simulink model "GUI_Simulaton"  (R2022b)
settings: Solver=ode1  StartTime=0.0  StopTime=3  FixedStep=20/(0.5*PWMclock)  RelTol=1e-3
InitFcn:
  | addpath('..\Library_Subsystems')
  | 
  | load('PWMLookUp.mat')
  | load('SimDefaultParam.mat')
  | 
  | samplerate = 10e-3;
  | samplerate_serial = 100e-3;
  | samplerate_udp = 100e-3;
  | 
  | fsw = 10000;
  | 
  | PWMclock = 100e6;
  | period = PWMclock/fsw/2;
model workspace (MAT data in the model file):
  DPWM0 = Simulink.Parameter
  DPWM0.Value.Du = [0.75 0.752642797452 0.755257258329 0.757843284196 0.760400777693 0.762929642529 0.765429783496 0.767901106464 0.77034351839 0.772756927317 0.775141242383 0.77749637382 ... (1024 elements, 1024x1)]
  DPWM0.Value.Dusec = [-0.5 -0.5 -0.5 -0.5 -0.5 -0.5 -0.5 -0.5 -0.5 -0.5 -0.5 -0.5 ... (1024 elements, 1024x1)]
  DPWM0.Value.Duclamp = [0 0 0 0 0 0 0 0 0 0 0 0 ... (1024 elements, 1024x1)]
  DPWM0.Value.Dv = [0 0.00531383198086 0.0106274638989 0.015940695699 0.0212533273409 0.0265651588071 0.03187599011 0.0371856212999 0.0424938524722 0.0478004837749 0.0531053154165 0.0584081476729 ... (1024 elements, 1024x1)]
  DPWM0.Value.Dvsec = [-0.5 -0.5 -0.5 -0.5 -0.5 -0.5 -0.5 -0.5 -0.5 -0.5 -0.5 -0.5 ... (1024 elements, 1024x1)]
  DPWM0.Value.Dvclamp = [0 0 0 0 0 0 0 0 0 0 0 0 ... (1024 elements, 1024x1)]
  DPWM0.Value.Dw = [0 0 0 0 0 0 0 0 0 0 0 0 ... (1024 elements, 1024x1)]
  DPWM0.Value.Dwsec = [-0.5 -0.5 -0.5 -0.5 -0.5 -0.5 -0.5 -0.5 -0.5 -0.5 -0.5 -0.5 ... (1024 elements, 1024x1)]
  DPWM0.Value.Dwclamp = [2 2 2 2 2 2 2 2 2 2 2 2 ... (1024 elements, 1024x1)]
  DPWM0.Value.Dufi = [12288 12331 12374 12417 12458 12500 12541 12581 12621 12661 12700 12739 ... (1024 elements, 1024x1)]
  DPWM0.Value.Dusecfi = [-8192 -8192 -8192 -8192 -8192 -8192 -8192 -8192 -8192 -8192 -8192 -8192 ... (1024 elements, 1024x1)]
  DPWM0.Value.Dvfi = [0 87 174 261 348 435 522 609 696 783 870 957 ... (1024 elements, 1024x1)]
  DPWM0.Value.Dvsecfi = [-8192 -8192 -8192 -8192 -8192 -8192 -8192 -8192 -8192 -8192 -8192 -8192 ... (1024 elements, 1024x1)]
  DPWM0.Value.Dwfi = [0 0 0 0 0 0 0 0 0 0 0 0 ... (1024 elements, 1024x1)]
  DPWM0.Value.Dwsecfi = [-8192 -8192 -8192 -8192 -8192 -8192 -8192 -8192 -8192 -8192 -8192 -8192 ... (1024 elements, 1024x1)]
  DPWM0.DataType = 'struct'
  DPWM0.Complexity = 'real'
  DPWM0.Dimensions = [1 1]
  DPWM1.Duclamp = [1 1 1 1 1 1 1 1 1 1 1 1 ... (1024 elements, 1024x1)]
  DPWM1.Dvclamp = [0 0 0 0 0 0 0 0 0 0 0 0 ... (1024 elements, 1024x1)]
  DPWM1.Dwclamp = [0 0 0 0 0 0 0 0 0 0 0 0 ... (1024 elements, 1024x1)]
  DPWM1.Dufi = [0 0 0 0 0 0 0 0 0 0 0 0 ... (1024 elements, 1024x1)]
  DPWM1.Dusecfi = [8192 8192 8192 8192 8192 8192 8192 8192 8192 8192 8192 8192 ... (1024 elements, 1024x1)]
  DPWM1.Dvfi = [-12288 -12244 -12200 -12155 -12110 -12065 -12019 -11972 -11925 -11878 -11830 -11782 ... (1024 elements, 1024x1)]
  DPWM1.Dvsecfi = [8192 8192 8192 8192 8192 8192 8192 8192 8192 8192 8192 8192 ... (1024 elements, 1024x1)]
  DPWM1.Dwfi = [-12288 -12331 -12374 -12417 -12458 -12500 -12541 -12581 -12621 -12661 -12700 -12739 ... (1024 elements, 1024x1)]
  DPWM1.Dwsecfi = [8192 8192 8192 8192 8192 8192 8192 8192 8192 8192 8192 8192 ... (1024 elements, 1024x1)]
  DPWM2.Duclamp = [1 1 1 1 1 1 1 1 1 1 1 1 ... (1024 elements, 1024x1)]
  DPWM2.Dvclamp = [0 0 0 0 0 0 0 0 0 0 0 0 ... (1024 elements, 1024x1)]
  DPWM2.Dwclamp = [0 0 0 0 0 0 0 0 0 0 0 0 ... (1024 elements, 1024x1)]
  DPWM2.Dufi = [0 0 0 0 0 0 0 0 0 0 0 0 ... (1024 elements, 1024x1)]
  DPWM2.Dusecfi = [8192 8192 8192 8192 8192 8192 8192 8192 8192 8192 8192 8192 ... (1024 elements, 1024x1)]
  DPWM2.Dvfi = [-12288 -12244 -12200 -12155 -12110 -12065 -12019 -11972 -11925 -11878 -11830 -11782 ... (1024 elements, 1024x1)]
  DPWM2.Dvsecfi = [8192 8192 8192 8192 8192 8192 8192 8192 8192 8192 8192 8192 ... (1024 elements, 1024x1)]
  DPWM2.Dwfi = [-12288 -12331 -12374 -12417 -12458 -12500 -12541 -12581 -12621 -12661 -12700 -12739 ... (1024 elements, 1024x1)]
  DPWM2.Dwsecfi = [8192 8192 8192 8192 8192 8192 8192 8192 8192 8192 8192 8192 ... (1024 elements, 1024x1)]
  DPWM3.Duclamp = [0 0 0 0 0 0 0 0 0 0 0 0 ... (1024 elements, 1024x1)]
  DPWM3.Dvclamp = [0 0 0 0 0 0 0 0 0 0 0 0 ... (1024 elements, 1024x1)]
  DPWM3.Dwclamp = [2 2 2 2 2 2 2 2 2 2 2 2 ... (1024 elements, 1024x1)]
  DPWM3.Dufi = [12288 12331 12374 12417 12458 12500 12541 12581 12621 12661 12700 12739 ... (1024 elements, 1024x1)]
  DPWM3.Dusecfi = [-8192 -8192 -8192 -8192 -8192 -8192 -8192 -8192 -8192 -8192 -8192 -8192 ... (1024 elements, 1024x1)]
  DPWM3.Dvfi = [0 87 174 261 348 435 522 609 696 783 870 957 ... (1024 elements, 1024x1)]
  DPWM3.Dvsecfi = [-8192 -8192 -8192 -8192 -8192 -8192 -8192 -8192 -8192 -8192 -8192 -8192 ... (1024 elements, 1024x1)]
  DPWM3.Dwfi = [0 0 0 0 0 0 0 0 0 0 0 0 ... (1024 elements, 1024x1)]
  DPWM3.Dwsecfi = [-8192 -8192 -8192 -8192 -8192 -8192 -8192 -8192 -8192 -8192 -8192 -8192 ... (1024 elements, 1024x1)]
  DPWMmax.Duclamp = [1 1 1 1 1 1 1 1 1 1 1 1 ... (1024 elements, 1024x1)]
  DPWMmax.Dvclamp = [0 0 0 0 0 0 0 0 0 0 0 0 ... (1024 elements, 1024x1)]
  DPWMmax.Dwclamp = [0 0 0 0 0 0 0 0 0 0 0 0 ... (1024 elements, 1024x1)]
  DPWMmax.Dufi = [0 0 0 0 0 0 0 0 0 0 0 0 ... (1024 elements, 1024x1)]
  DPWMmax.Dusecfi = [8192 8192 8192 8192 8192 8192 8192 8192 8192 8192 8192 8192 ... (1024 elements, 1024x1)]
  DPWMmax.Dvfi = [-12288 -12244 -12200 -12155 -12110 -12065 -12019 -11972 -11925 -11878 -11830 -11782 ... (1024 elements, 1024x1)]
  DPWMmax.Dvsecfi = [8192 8192 8192 8192 8192 8192 8192 8192 8192 8192 8192 8192 ... (1024 elements, 1024x1)]
  DPWMmax.Dwfi = [-12288 -12331 -12374 -12417 -12458 -12500 -12541 -12581 -12621 -12661 -12700 -12739 ... (1024 elements, 1024x1)]
  DPWMmax.Dwsecfi = [8192 8192 8192 8192 8192 8192 8192 8192 8192 8192 8192 8192 ... (1024 elements, 1024x1)]
  DPWMmin.Duclamp = [0 0 0 0 0 0 0 0 0 0 0 0 ... (1024 elements, 1024x1)]
  DPWMmin.Dvclamp = [0 0 0 0 0 0 0 0 0 0 0 0 ... (1024 elements, 1024x1)]
  DPWMmin.Dwclamp = [2 2 2 2 2 2 2 2 2 2 2 2 ... (1024 elements, 1024x1)]
  DPWMmin.Dufi = [12288 12331 12374 12417 12458 12500 12541 12581 12621 12661 12700 12739 ... (1024 elements, 1024x1)]
  DPWMmin.Dusecfi = [-8192 -8192 -8192 -8192 -8192 -8192 -8192 -8192 -8192 -8192 -8192 -8192 ... (1024 elements, 1024x1)]
  DPWMmin.Dvfi = [0 87 174 261 348 435 522 609 696 783 870 957 ... (1024 elements, 1024x1)]
  DPWMmin.Dvsecfi = [-8192 -8192 -8192 -8192 -8192 -8192 -8192 -8192 -8192 -8192 -8192 -8192 ... (1024 elements, 1024x1)]
  DPWMmin.Dwfi = [0 0 0 0 0 0 0 0 0 0 0 0 ... (1024 elements, 1024x1)]
  DPWMmin.Dwsecfi = [-8192 -8192 -8192 -8192 -8192 -8192 -8192 -8192 -8192 -8192 -8192 -8192 ... (1024 elements, 1024x1)]
  SPWM.Dufi = [8192 8192 8191 8191 8190 8188 8186 8184 8182 8180 8177 8173 ... (1024 elements, 1024x1)]
  SPWM.Dvfi = [-4096 -4052 -4009 -3965 -3921 -3876 -3832 -3788 -3743 -3698 -3653 -3608 ... (1024 elements, 1024x1)]
  SPWM.Dwfi = [-4096 -4139 -4183 -4226 -4269 -4312 -4354 -4397 -4439 -4481 -4523 -4565 ... (1024 elements, 1024x1)]
  SVPWM.Dufi = [6144 6166 6187 6208 6229 6250 6270 6291 6311 6330 6350 6369 ... (1024 elements, 1024x1)]
  SVPWM.Dvfi = [-6144 -6079 -6013 -5947 -5881 -5815 -5748 -5681 -5614 -5547 -5480 -5412 ... (1024 elements, 1024x1)]
  SVPWM.Dwfi = [-6144 -6166 -6187 -6208 -6229 -6250 -6270 -6291 -6311 -6330 -6350 -6369 ... (1024 elements, 1024x1)]
  THISPWM.Dufi = [6823 6823 6823 6823 6824 6825 6826 6827 6828 6829 6831 6832 ... (1024 elements, 1024x1)]
  THISPWM.Dvfi = [-5465 -5421 -5377 -5332 -5286 -5240 -5193 -5145 -5097 -5049 -4999 -4949 ... (1024 elements, 1024x1)]
  THISPWM.Dwfi = [-5465 -5508 -5551 -5593 -5634 -5675 -5715 -5755 -5794 -5832 -5869 -5906 ... (1024 elements, 1024x1)]
  THISPWM.THIfi = [1369 1369 1368 1367 1366 1363 1361 1358 1354 1350 1346 1341 ... (1024 elements, 1024x1)]
undefined symbols (not defined in the file): ASCMode, LoadL, LoadR, ModIdx, poshillhold, possync, PWMMode, Speed, Vdc
libraries: spsParallelRLCBranchLib x6, spsControlledVoltageSourceLib x3, spsCurrentMeasurementLib x3, spsVariableInductorLib x3, spsVariableResistorLib x3, simulink x2, spspowerguiLib x1
settings Model: SimulationMode=rapid-accelerator  TunableVars=DPWM0,DPWM2,DPWM3,DPWMmax,DPWMmin,SPWM,SVPWM,THISPWM  TunableVarsStorageClass=Auto,Auto,Auto,Auto,Auto,Auto,Auto,Auto  TunableVarsTypeQualifier=,,,,,,,  Creator=ReiterTo  LastModifiedBy=ReiterTo
settings SolverCC: AlgebraicLoopSolver=TrustRegion  PositivePriorityOrder=on  AutoInsertRateTranBlk=on
settings DataIOCC: MaxDataPoints=10000  SaveFormat=Array  InspectSignalLogs=on
settings OptimizationCC: EnhancedBackFolding=on  StrengthReduction=on  PassReuseOutputArgsThreshold=0  EfficientFloat2IntCast=on  MaxStackSize=64  OptimizeBlockOrder=speed  OptimizationPriority=Speed  MultiThreadedLoops=on
settings DebuggingCC: ParameterOverflowMsg=none  ParameterPrecisionLossMsg=none  ParameterTunabilityLossMsg=error
settings HardwareCC: ProdBitPerPointer=32  ProdBitPerSizeT=32  ProdBitPerPtrDiffT=32  ProdLargestAtomicInteger=Long  ProdLargestAtomicFloat=Double  ProdWordSize=32  ProdHWDeviceType=ARM Compatible->ARM Cortex  TargetBitPerPointer=64  TargetBitPerSizeT=64  TargetBitPerPtrDiffT=64  TargetLongLongMode=on  TargetIntDivRoundTo=Zero  TargetEndianess=LittleEndian  TargetWordSize=64  TargetHWDeviceType=MATLAB Host  ProdEqTarget=off
settings SFSimCC: MATLABDynamicMemAlloc=off
settings RTWCC: Description=Rapid Simulation Target  SystemTargetFile=rsim.tlc  TemplateMakefile=rsim_default_tmf  Toolchain=Arduino ARM  BuildConfiguration=Faster Runs  CheckMdlBeforeBuild=Warning
settings CodeAppCC: ForceParamTrailComments=on  OperatorAnnotations=on
settings RSimTargetCC: TargetLangStandard=C99 (ISO)  OptimizeReductions=off

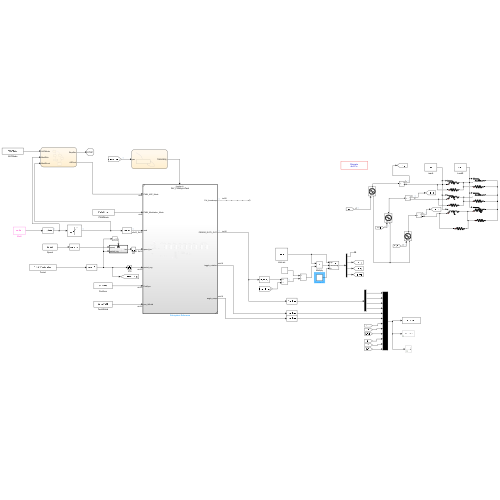
[thumbnail: Simulink's stored preview of the top-level diagram]
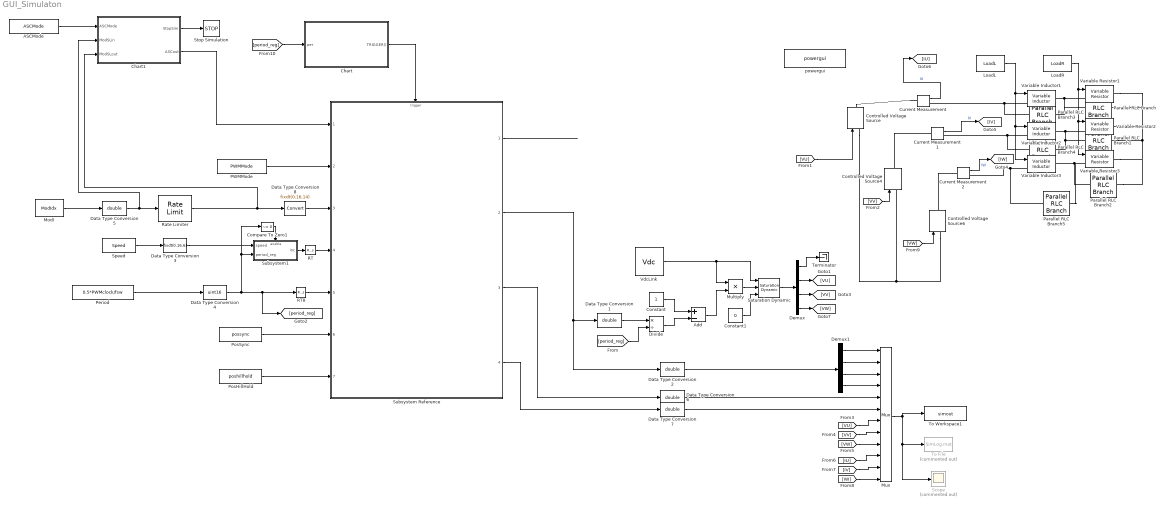
== system GUI_Simulaton ==
  ASCMode : Constant  Value=ASCMode  OutDataTypeStr=uint8
  Add : Sum  Inputs=+-
  Chart : Stateflow chart  TreatAsAtomicUnit=on
  Chart1 : Stateflow chart  TreatAsAtomicUnit=on
  Compare To Zero1 : simulink/Logic and Bit Operations/Compare To Zero  relop=~=  OutDataTypeStr=boolean
  Constant : Constant
  Constant1 : Constant  Value=0
  Controlled Voltage Source : spsControlledVoltageSourceLib/Controlled Voltage Source  Initialize=on  Source_Type=DC  Amplitude=0  Phase=0  Frequency=0  Measurements=None
  Controlled Voltage Source4 : spsControlledVoltageSourceLib/Controlled Voltage Source  Initialize=on  Source_Type=DC  Amplitude=0  Phase=0  Frequency=0  Measurements=None
  Controlled Voltage Source6 : spsControlledVoltageSourceLib/Controlled Voltage Source  Initialize=on  Source_Type=DC  Amplitude=0  Phase=0  Frequency=0  Measurements=None
  Current Measurement : spsCurrentMeasurementLib/Current Measurement  PhasorSimulation=off  OutputType=Complex  PSBequivalent=0
  Current Measurement1 : spsCurrentMeasurementLib/Current Measurement  PhasorSimulation=off  OutputType=Complex  PSBequivalent=0
  Current Measurement2 : spsCurrentMeasurementLib/Current Measurement  PhasorSimulation=off  OutputType=Complex  PSBequivalent=0
  Data Type Conversion{1..2,5..7} (5 alike) : DataTypeConversion  OutDataTypeStr=double  SaturateOnIntegerOverflow=off  RndMeth=Floor
  Data Type Conversion3 : DataTypeConversion  OutDataTypeStr=fixdt(0,16,6)  SaturateOnIntegerOverflow=off  RndMeth=Floor
  Data Type Conversion4 : DataTypeConversion  OutDataTypeStr=uint16  SaturateOnIntegerOverflow=off  RndMeth=Floor
  Data Type Conversion8 : DataTypeConversion  OutDataTypeStr=fixdt(0,16,14)  SaturateOnIntegerOverflow=off  RndMeth=Floor
  Demux : Demux
  Demux1 : Demux
  Divide : Product  Inputs=*/  OutDataTypeStr=double  RndMeth=Simplest
  LoadL : Constant  Value=LoadL  OutDataTypeStr=double
  LoadR : Constant  Value=LoadR  OutDataTypeStr=double
  ModI : Constant  Value=ModIdx  OutDataTypeStr=double
  Multiply : Product  Inputs=**  OutDataTypeStr=double  RndMeth=Simplest
  Mux : Mux  Inputs=12
  PWMMode : Constant  Value=PWMMode  OutDataTypeStr=uint8
  Parallel RLC Branch{,1..5} (6 alike) : spsParallelRLCBranchLib/Parallel RLC Branch  LConnTagsString=a  RConnTagsString=__new0  BranchType=R  Resistance=10e3  Inductance=1e-3  SetiL0=off  InitialCurrent=0  Capacitance=1e-6  Setx0=off  InitialVoltage=0  Measurements=None
  Period : Constant  Value=0.5*PWMclock/fsw  OutDataTypeStr=uint16
  PosHillHold : Constant  Value=poshillhold  OutDataTypeStr=uint16
  PosSync : Constant  Value=possync  OutDataTypeStr=uint16
  RT : RateTransition  Deterministic=off
  RT8 : RateTransition  Deterministic=off
  Rate Limiter : RateLimiter  RisingSlewLimit=2  FallingSlewLimit=-2  SampleTimeMode=inherited
  Saturation Dynamic : simulink/Discontinuities/Saturation Dynamic  OutMin=[]  OutMax=[]  OutDataTypeStr=Inherit: Same as second input  OutDataType=fixdt(1, 16)  OutScaling=2^-10  DoSatur=off
  Scope : Scope  Commented=on
  Speed : Constant  Value=Speed  OutDataTypeStr=double
  Stop Simulation : Stop
  Subsystem Reference : Subsystem  ReferencedSubsystem=INV_PWMsyncTask
  Subsystem1 : Subsystem
  Terminator : Terminator
  To File : ToFile  Commented=on  Filename=SimLog.mat  MatrixName=Logdata
  To Workspace1 : ToWorkspace  VariableName=simout  SampleTime=-1
  Variable Inductor1 : spsVariableInductorLib/Variable Inductor  methode=Backward Euler  Labsmin=100e-9  Initialize=on  iL0=0  L0=100e-9  Vl0=0
      settings: LibrarySourceBlock=sps_lib/Passives/Variable Inductor
  Variable Inductor2 : spsVariableInductorLib/Variable Inductor  methode=Backward Euler  Labsmin=100e-9  Initialize=on  iL0=0  L0=100e-9  Vl0=0
      settings: LibrarySourceBlock=sps_lib/Passives/Variable Inductor
  Variable Inductor3 : spsVariableInductorLib/Variable Inductor  methode=Backward Euler  Labsmin=100e-9  Initialize=on  iL0=0  L0=100e-9  Vl0=0
      settings: LibrarySourceBlock=sps_lib/Passives/Variable Inductor
  Variable Resistor1 : spsVariableResistorLib/Variable Resistor  Rabsmin=1e-3
      settings: LibrarySourceBlock=sps_lib/Passives/Variable Resistor
  Variable Resistor2 : spsVariableResistorLib/Variable Resistor  Rabsmin=1e-3
      settings: LibrarySourceBlock=sps_lib/Passives/Variable Resistor
  Variable Resistor3 : spsVariableResistorLib/Variable Resistor  Rabsmin=1e-3
      settings: LibrarySourceBlock=sps_lib/Passives/Variable Resistor
  VdcLink : Constant  Value=Vdc  OutDataTypeStr=double
  powergui : spspowerguiLib/powergui  Priority=1  SimulationMode=Discrete  SampleTime=20/(0.5*PWMclock)  frequency=60  Iterations=50  frequencyindice=0  Pbase=100e6  ErrMax=1e-4  UnitsV=kV  UnitsW=MW  buscounter=0  FunctionMessages=off  echomessages=off  EnableUseOfTLC=off  CurrentSourceSwitches=off  DisableSnubberDevices=off  DisableRonSwitches=off  DisableVfSwitches=off  DisplayEquations=off  AutomaticDiscreteSolvers=off  SolverType=Tustin/Backward Euler (TBE)  Interpol=off  ExternalGateDelay=off  methode=off  Ts=100  x0status=blocks  SPID=on  SwTol=0  HookPort=off  NonlinearTolerance=1e-4  nMaxIteration=100  ContinueOnMaxIteration=off  RestoreLinks=warning  ResistiveCurrentMeasurement=off  Frange=[0:2:500]  Ylog=off  Xlog=on  ShowGrid=off  save=off  variable=ZData  structure=0  ZoomFFT=off  StartTime=0.0  cycles=1  DisplayStyle=1  fundamental=60  FreqAxis=off  MaxFrequency=1000  frequencyindicesteady=1  RmsSteady=1  display=off
  wires:
  Current Measurement1/1 -> [IV]  "IV"
  Mux/1 -> To Workspace1/1, Scope/1, To File/1
  Current Measurement2/1 -> [IW]  "IW"
  Current Measurement/1 -> [IU]  "IU"
  PosSync/1 -> Subsystem Reference/6
  PosHillHold/1 -> Subsystem Reference/7
  RT8/1 -> Subsystem Reference/5
  RT/1 -> Subsystem Reference/4
  Data Type Conversion3/1 -> Subsystem1/1(speed)
  Subsystem1/1(inc) -> RT/1
  Compare To Zero1/1 -> Subsystem1/Enable
  Data Type Conversion4/1 -> Compare To Zero1/1, Subsystem1/2(period_reg), [period_reg], RT8/1
  Speed/1 -> Data Type Conversion3/1
  Data Type Conversion1/1 -> Divide/1
  [period_reg] -> Divide/2
  VdcLink/1 -> Saturation Dynamic/1, Multiply/1
  [VU] -> Controlled Voltage Source/1
  [VW] -> Controlled Voltage Source6/1
  [VV] -> Controlled Voltage Source4/1
  Subsystem Reference/2 -> Data Type Conversion2/1, Data Type Conversion1/1
  Data Type Conversion2/1 -> Demux1/1
  Data Type Conversion5/1 -> Rate Limiter/1, Chart1/2(ModSLin)
  LoadL/1 -> Variable Inductor3/1, Variable Inductor2/1, Variable Inductor1/1
  LoadR/1 -> Variable Resistor3/1, Variable Resistor2/1, Variable Resistor1/1
  Demux1/1 -> Mux/1
  Demux1/2 -> Mux/2
  Demux1/3 -> Mux/3
  Demux1/4 -> Mux/4
  Subsystem Reference/3 -> Data Type Conversion6/1
  Subsystem Reference/4 -> Data Type Conversion7/1
  [VU] -> Mux/7
  [VV] -> Mux/8
  [VW] -> Mux/9
  [IU] -> Mux/10
  [IV] -> Mux/11
  [IW] -> Mux/12
  Data Type Conversion6/1 -> Mux/5
  Data Type Conversion7/1 -> Mux/6
  Demux/4 -> [VW]
  Demux/3 -> [VV]
  Demux/2 -> [VU]
  Demux/1 -> Terminator/1
  Chart/1(TRIGGER()) -> Subsystem Reference/Trigger
  [period_reg] -> Chart/1(per)
  Subsystem Reference/1 -> ?
  Rate Limiter/1 -> Chart1/3(ModSLout), Data Type Conversion8/1
  Data Type Conversion8/1 -> Subsystem Reference/3
  Chart1/1(StopSim) -> Stop Simulation/1
  Period/1 -> Data Type Conversion4/1
  Chart1/2(ASCout) -> Subsystem Reference/1
  ASCMode/1 -> Chart1/1(ASCMode)
  Constant/1 -> Add/1
  Divide/1 -> Add/2
  Add/1 -> Multiply/2
  ModI/1 -> Data Type Conversion5/1
  PWMMode/1 -> Subsystem Reference/2
  Multiply/1 -> Saturation Dynamic/2
  Saturation Dynamic/1 -> Demux/1
  Constant1/1 -> Saturation Dynamic/3
  connections:
  Controlled Voltage Source/LConn1 -- Controlled Voltage Source6/LConn1 -- Controlled Voltage Source4/LConn1
  Current Measurement/LConn1 -- Controlled Voltage Source/RConn1
  Current Measurement2/LConn1 -- Controlled Voltage Source6/RConn1
  Controlled Voltage Source4/RConn1 -- Current Measurement1/LConn1
  Variable Inductor1/LConn1 -- Parallel RLC Branch3/LConn1 -- Current Measurement/RConn1
  Variable Resistor1/LConn1 -- Parallel RLC Branch3/RConn1 -- Parallel RLC Branch/LConn1 -- Variable Inductor1/RConn1
  Variable Resistor2/LConn1 -- Parallel RLC Branch4/RConn1 -- Parallel RLC Branch1/LConn1 -- Variable Inductor2/RConn1
  Variable Resistor3/LConn1 -- Parallel RLC Branch5/RConn1 -- Parallel RLC Branch2/LConn1 -- Variable Inductor3/RConn1
  Variable Inductor3/LConn1 -- Parallel RLC Branch5/LConn1 -- Current Measurement2/RConn1
  Variable Inductor2/LConn1 -- Parallel RLC Branch4/LConn1 -- Current Measurement1/RConn1
  Variable Resistor1/RConn1 -- Parallel RLC Branch/RConn1 -- Parallel RLC Branch2/RConn1 -- Variable Resistor3/RConn1 -- Parallel RLC Branch1/RConn1 -- Variable Resistor2/RConn1

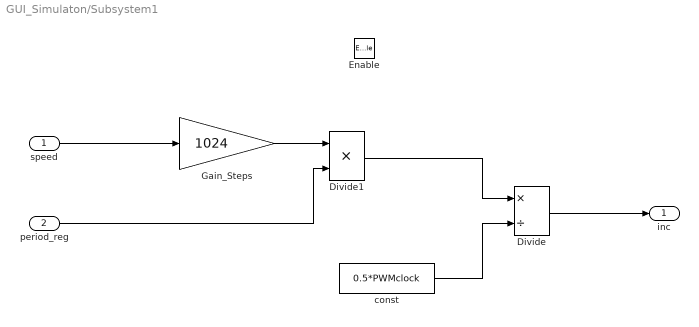
== system GUI_Simulaton/Subsystem1 ==
  speed : Inport
  period_reg : Inport  Port=2
  Enable : EnablePort
  Divide : Product  Inputs=*/  OutDataTypeStr=fixdt(0,32,16)  RndMeth=Simplest
  Divide1 : Product  Inputs=**  OutDataTypeStr=uint32  RndMeth=Simplest
  Gain_Steps : Gain  Gain=1024  ParamDataTypeStr=int32  OutDataTypeStr=uint32  RndMeth=Simplest  LockScale=on
  const : Constant  Value=0.5*PWMclock  OutDataTypeStr=uint32
  inc : Outport
  wires:
  speed/1 -> Gain_Steps/1
  const/1 -> Divide/2
  period_reg/1 -> Divide1/2
  Gain_Steps/1 -> Divide1/1
  Divide1/1 -> Divide/1
  Divide/1 -> inc/1

== stateflow chart GUI_Simulaton/Chart1 ==
  state Select
  state RunSim
  state RunSimASC
  state RunSimtoSteady
  state SimASC
    en: ASCout=ASCMode;
  state StopSim
    en:StopSim = 1;
  (default) -> Select
  Select -> RunSim [order 1] : [ASCMode==0]
  Select -> RunSimASC [order 2]
  RunSim -> RunSimtoSteady : [ModSLin==ModSLout]
  RunSimASC -> (junction 140) : [ModSLin==ModSLout]
  (junction 140) -> SimASC : [after(0.3,sec)]
  RunSimtoSteady -> StopSim : [after(0.3,sec)]
  SimASC -> StopSim : [after(0.3,sec)]
  data: ASCMode input; ModSLin input; ModSLout input; StopSim output boolean =0; ASCout output uint8 =uint8(0)

== stateflow chart GUI_Simulaton/Chart ==
  state Trigger_State
    en: send(TRIGGER);
  (default) -> Trigger_State
  Trigger_State -> Trigger_State : [after((per/20),tick)]
  data: per input
  events: TRIGGER output FUNCTION_CALL_EVENT
